simulink model "AT_power_supply"  (R2017a)
settings: Solver=VariableStepDiscrete  StartTime=0.0  StopTime=10.0  MaxStep=1e-4  RelTol=1e-3
model workspace (MAT data in the model file):
  C = [1.22730985268e-11  -9.79032554766e-13  -3.3876063565e-12  -2.00231039085e-12  -3.89359662643e-13  -1.2256864147e-12; -9.79032554766e-13  8.8541386421e-12  -3.48812783487e-12  -6.7988448902e-13  -2.32120771084e-13  -3.75147725397e-13; -3.3876063565e-12  -3.48812783487e-12  5.05683717303e-11  -4.82296810228e-13  -4.29846925887e-14  -1.14861569096e-12; -2.00231039085e-12  -6.7988448902e-13  -4.82296810228e-13  1.2217542164e-11  -1.06668598412e-12  -3.29793326195e-12; -3.89359662643e-13  -2.32120771084e-13  -4.29846925887e-14  -1.06668598412e-12  8.80500883356e-12  -3.55300206066e-12; -1.2256864147e-12  -3.75147725397e-13  -1.14861569096e-12  -3.29793326195e-12  -3.55300206066e-12  5.14882367603e-11]
  L = [0.00187555920474  0.00102764893826  0.00103076007408  0.00104087588335  0.000916441165262  0.00094103834573; 0.00102764893826  0.00220486482933  0.0010632014985  0.000914578394203  0.000842167961305  0.000853030250716; 0.00103076007408  0.0010632014985  0.00138127517435  0.000946699228346  0.000884811406268  0.000952474726801; 0.00104087588335  0.000914578394203  0.000946699228346  0.0018795120154  0.0010307312193  0.00103493155019; 0.000916441165262  0.000842167961305  0.000884811406268  0.0010307312193  0.00220867896719  0.00106461641191; 0.00094103834573  0.000853030250716  0.000952474726801  0.00103493155019  0.00106461641191  0.00136582310124]
  X = [0.589224301899  0.322845435491  0.323822827633  0.327000802842  0.287908483223  0.295635915369; 0.322845435491  0.692678715  0.334014601697  0.287323276436  0.264574868032  0.267987356894; 0.323822827633  0.334014601697  0.433940394034  0.297414334093  0.277971701374  0.299228760445; 0.327000802842  0.287323276436  0.297414334093  0.590466113991  0.323813762639  0.325133335506; 0.287908483223  0.264574868032  0.277971701374  0.323813762639  0.693876961748  0.334459109856; 0.295635915369  0.267987356894  0.299228760445  0.325133335506  0.334459109856  0.429085982097]
libraries: powerlib x20
settings Model: Creator=Administrator  LastModifiedBy=Administrator
settings DebuggingCC: UnconnectedInputMsg=none  UnconnectedOutputMsg=none  UnconnectedLineMsg=none

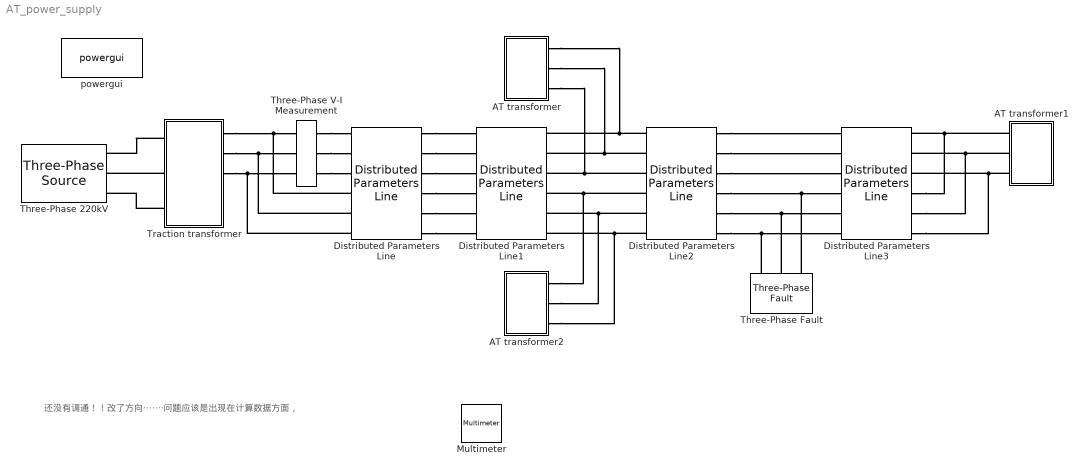
== system AT_power_supply ==
  note: 还没有调通！！改了方向·······问题应该是出现在计算数据方面，
  AT transformer : Subsystem
  AT transformer1 : Subsystem
  AT transformer2 : Subsystem
  Distributed Parameters Line : powerlib/Elements/Distributed Parameters Line  Phases=6  Frequency=50  Resistance=X  Inductance=L  Capacitance=C  Length=100  x1=[0 0 0 0; 0.0001244 0 0 0; 0.0002488 0 0 0; 0.0003733 0 0 0; 0.0004977 0 0 0; 0.0006221 0 0 0]  x2=[0 0 0 0; 0.0001244 0 0 0; 0.0002488 0 0 0; 0.0003733 0 0 0; 0.0004977 0 0 0; 0.0006221 0 0 0]  x3=[0 0 0 0; 0.0001244 0 0 0; 0.0002488 0 0 0; 0.0003733 0 0 0; 0.0004977 0 0 0; 0.0006221 0 0 0]  x4=[0 0 0 0; 0.0001244 0 0 0; 0.0002488 0 0 0; 0.0003733 0 0 0; 0.0004977 0 0 0; 0.0006221 0 0 0]  x5=0  V1=ones(3,3)  V2=ones(3,3)  I1=ones(3,3)  I2=ones(3,3)  nHarmo=1  Measurements=Phase-to-ground voltages
      settings: SourceProductName=Simscape Power Systems
  Distributed Parameters Line1 : powerlib/Elements/Distributed Parameters Line  Phases=6  Frequency=50  Resistance=X  Inductance=L  Capacitance=C  Length=10  x1=[0 0 0 0; 0.0001244 0 0 0; 0.0002488 0 0 0; 0.0003733 0 0 0; 0.0004977 0 0 0; 0.0006221 0 0 0]  x2=[0 0 0 0; 0.0001244 0 0 0; 0.0002488 0 0 0; 0.0003733 0 0 0; 0.0004977 0 0 0; 0.0006221 0 0 0]  x3=[0 0 0 0; 0.0001244 0 0 0; 0.0002488 0 0 0; 0.0003733 0 0 0; 0.0004977 0 0 0; 0.0006221 0 0 0]  x4=[0 0 0 0; 0.0001244 0 0 0; 0.0002488 0 0 0; 0.0003733 0 0 0; 0.0004977 0 0 0; 0.0006221 0 0 0]  x5=0  V1=ones(3,3)  V2=ones(3,3)  I1=ones(3,3)  I2=ones(3,3)  nHarmo=1  Measurements=None
      settings: SourceProductName=Simscape Power Systems
  Distributed Parameters Line2 : powerlib/Elements/Distributed Parameters Line  Phases=6  Frequency=50  Resistance=X  Inductance=L  Capacitance=C  Length=10  x1=[0 0 0 0; 0.0001244 0 0 0; 0.0002488 0 0 0; 0.0003733 0 0 0; 0.0004977 0 0 0; 0.0006221 0 0 0]  x2=[0 0 0 0; 0.0001244 0 0 0; 0.0002488 0 0 0; 0.0003733 0 0 0; 0.0004977 0 0 0; 0.0006221 0 0 0]  x3=[0 0 0 0; 0.0001244 0 0 0; 0.0002488 0 0 0; 0.0003733 0 0 0; 0.0004977 0 0 0; 0.0006221 0 0 0]  x4=[0 0 0 0; 0.0001244 0 0 0; 0.0002488 0 0 0; 0.0003733 0 0 0; 0.0004977 0 0 0; 0.0006221 0 0 0]  x5=0  V1=ones(3,3)  V2=ones(3,3)  I1=ones(3,3)  I2=ones(3,3)  nHarmo=1  Measurements=None
      settings: SourceProductName=Simscape Power Systems
  Distributed Parameters Line3 : powerlib/Elements/Distributed Parameters Line  Phases=6  Frequency=50  Resistance=X  Inductance=L  Capacitance=C  Length=10  x1=[0 0 0 0; 0.0001244 0 0 0; 0.0002488 0 0 0; 0.0003733 0 0 0; 0.0004977 0 0 0; 0.0006221 0 0 0]  x2=[0 0 0 0; 0.0001244 0 0 0; 0.0002488 0 0 0; 0.0003733 0 0 0; 0.0004977 0 0 0; 0.0006221 0 0 0]  x3=[0 0 0 0; 0.0001244 0 0 0; 0.0002488 0 0 0; 0.0003733 0 0 0; 0.0004977 0 0 0; 0.0006221 0 0 0]  x4=[0 0 0 0; 0.0001244 0 0 0; 0.0002488 0 0 0; 0.0003733 0 0 0; 0.0004977 0 0 0; 0.0006221 0 0 0]  x5=0  V1=ones(3,3)  V2=ones(3,3)  I1=ones(3,3)  I2=ones(3,3)  nHarmo=1  Measurements=None
      settings: SourceProductName=Simscape Power Systems
  Multimeter : powerlib/Measurements/Multimeter  PhasorSimulation=off  OutputType=Complex  sel=1  L=1  Gain=0  yselected={}  PSBOutputType=1  PSBequivalent=0  AxesSetting=[0,0.1,-100,100]  Display=0  SavedBlockNames=-11
  Three-Phase V-I Measurement : powerlib/Measurements/Three-Phase V-I Measurement  VoltageMeasurement=phase-to-ground  SetLabelV=on  LabelV=Vabc  Vpu=off  VpuLL=off  CurrentMeasurement=yes  SetLabelI=on  LabelI=Iabc  Ipu=off  Pbase=100e6  Vbase=500e3  OutputType=Complex  PhasorSimulation=off  PSBequivalent=0
  Three-Phase 220kV : powerlib/Electrical Sources/Three-Phase Source  InternalConnection=Yg  VoltagePhases=off  Voltage=220e3  PhaseAngle=0  Voltage_phases=[25e3 25e3 25e3]/sqrt(3)  PhaseAngles_phases=[0 -120 +120]  Frequency=50  NonIdealSource=on  SpecifyImpedance=on  Resistance=0.8929  Inductance=16.58e-3  ShortCircuitLevel=4e9  BaseVoltage=220e3  XRratio=16  BusType=swing  Pref=10e3  Qref=0  Prefabc=[10e3, 10e3, 10e3]  Qrefabc=[0, 0, 0]  Qmin=-inf  Qmax=inf
  Three-Phase Fault : powerlib/Elements/Three-Phase Fault  InitialStates=0  FaultA=on  FaultB=off  FaultC=off  GroundFault=on  SwitchTimes="[1/60  5/60]"  External=off  SwitchStatus=NaN  FaultResistance=0.001  GroundResistance=0.01  SnubberResistance=1e6  SnubberCapacitance=inf  Measurements=None
  Traction transformer : Subsystem
  powergui : powerlib/powergui  Priority=1  SimulationMode=Continuous  SampleTime=1e-6  frequency=60  Iterations=50  frequencyindice=60  Pbase=100e6  ErrMax=1e-4  UnitsV=kV  UnitsW=MW  buscounter=0  FunctionMessages=off  echomessages=off  EnableUseOfTLC=off  CurrentSourceSwitches=off  DisableSnubberDevices=off  DisableRonSwitches=off  DisableVfSwitches=off  DisplayEquations=off  SolverType=Tustin/Backward Euler (TBE)  Interpol=off  ExternalGateDelay=off  methode=off  Ts=100  x0status=blocks  SPID=on  SwTol=0  HookPort=off  RestoreLinks=warning  ResistiveCurrentMeasurement=off  Frange=[0:2:500]  Ylog=off  Xlog=on  ShowGrid=off  save=off  variable=ZData  structure=0  ZoomFFT=off  StartTime=0.0  cycles=1  DisplayStyle=1  fundamental=60  FreqAxis=off  MaxFrequency=1000  frequencyindicesteady=1  RmsSteady=1  display=off
  connections:
  Traction transformer/LConn2 -- Three-Phase 220kV/RConn2
  Traction transformer/LConn1 -- Three-Phase 220kV/RConn1
  Traction transformer/LConn3 -- Three-Phase 220kV/RConn3
  Distributed Parameters Line/RConn1 -- Distributed Parameters Line1/LConn1
  Distributed Parameters Line/RConn2 -- Distributed Parameters Line1/LConn2
  Distributed Parameters Line/RConn3 -- Distributed Parameters Line1/LConn3
  Distributed Parameters Line/RConn4 -- Distributed Parameters Line1/LConn4
  Distributed Parameters Line/RConn5 -- Distributed Parameters Line1/LConn5
  Distributed Parameters Line/RConn6 -- Distributed Parameters Line1/LConn6
  Distributed Parameters Line2/LConn1 -- AT transformer/RConn1 -- Distributed Parameters Line1/RConn1
  Distributed Parameters Line2/LConn2 -- AT transformer/RConn2 -- Distributed Parameters Line1/RConn2
  Distributed Parameters Line2/LConn3 -- AT transformer/RConn3 -- Distributed Parameters Line1/RConn3
  Distributed Parameters Line2/LConn4 -- AT transformer2/RConn1 -- Distributed Parameters Line1/RConn4
  Distributed Parameters Line2/LConn5 -- AT transformer2/RConn2 -- Distributed Parameters Line1/RConn5
  Distributed Parameters Line2/LConn6 -- AT transformer2/RConn3 -- Distributed Parameters Line1/RConn6
  Distributed Parameters Line2/RConn1 -- Distributed Parameters Line3/LConn1
  Distributed Parameters Line2/RConn2 -- Distributed Parameters Line3/LConn2
  Distributed Parameters Line2/RConn3 -- Distributed Parameters Line3/LConn3
  Distributed Parameters Line2/RConn4 -- Three-Phase Fault/LConn1 -- Distributed Parameters Line3/LConn4
  Distributed Parameters Line2/RConn5 -- Three-Phase Fault/LConn2 -- Distributed Parameters Line3/LConn5
  Distributed Parameters Line2/RConn6 -- Three-Phase Fault/LConn3 -- Distributed Parameters Line3/LConn6
  AT transformer1/RConn1 -- Distributed Parameters Line3/RConn4 -- Distributed Parameters Line3/RConn1
  AT transformer1/RConn2 -- Distributed Parameters Line3/RConn5 -- Distributed Parameters Line3/RConn2
  AT transformer1/RConn3 -- Distributed Parameters Line3/RConn6 -- Distributed Parameters Line3/RConn3
  Traction transformer/RConn1 -- Distributed Parameters Line/LConn4 -- Three-Phase V-I Measurement/LConn1
  Traction transformer/RConn2 -- Distributed Parameters Line/LConn5 -- Three-Phase V-I Measurement/LConn2
  Traction transformer/RConn3 -- Distributed Parameters Line/LConn6 -- Three-Phase V-I Measurement/LConn3
  Three-Phase V-I Measurement/RConn1 -- Distributed Parameters Line/LConn1
  Three-Phase V-I Measurement/RConn2 -- Distributed Parameters Line/LConn2
  Three-Phase V-I Measurement/RConn3 -- Distributed Parameters Line/LConn3

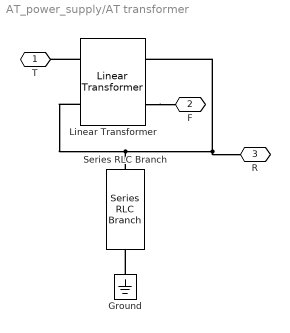
== system AT_power_supply/AT transformer ==
  Ground : powerlib/Elements/Ground  LConnTagsString=a
  Linear Transformer : powerlib/Elements/Linear Transformer  UNITS=pu  NominalPower=[ 32e6 50 ]  winding1="[ 27.5e3  0.002  0.08 ]"  winding2="[ 27.5e3  0.002  0.08 ]"  ThreeWindings=off  winding3=[ 315e3 0.002 0.08 ]  RmLm=[ 500 500 ]  Measurements=All voltages and currents  DataType=off
  Series RLC Branch : powerlib/Elements/Series RLC Branch  LConnTagsString=__new0  RConnTagsString=__new0  BranchType=R  Resistance=0.42  Inductance=1e-3  SetiL0=off  InitialCurrent=0  Capacitance=1e-6  Setx0=off  InitialVoltage=0  Measurements=None
  T : PMIOPort  Port=1  Side=Right
  F : PMIOPort  Port=2  Side=Right
  R : PMIOPort  Port=3  Side=Right
  connections:
  Linear Transformer/RConn2 -- F/RConn1
  Linear Transformer/LConn1 -- T/RConn1
  Ground/LConn1 -- Series RLC Branch/RConn1
  Linear Transformer/LConn2 -- Series RLC Branch/LConn1 -- R/RConn1 -- Linear Transformer/RConn1

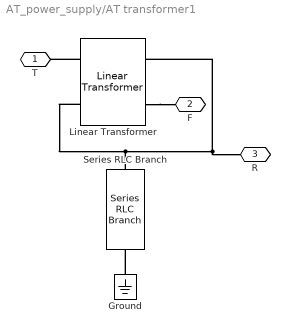
== system AT_power_supply/AT transformer1 ==
  Ground : powerlib/Elements/Ground  LConnTagsString=a
  Linear Transformer : powerlib/Elements/Linear Transformer  UNITS=pu  NominalPower=[ 32e6 50 ]  winding1="[ 27.5e3  0.002  0.08 ]"  winding2="[ 27.5e3  0.002  0.08 ]"  ThreeWindings=off  winding3=[ 315e3 0.002 0.08 ]  RmLm=[ 500 500 ]  Measurements=All voltages and currents  DataType=off
  Series RLC Branch : powerlib/Elements/Series RLC Branch  LConnTagsString=__new0  RConnTagsString=__new0  BranchType=R  Resistance=0.42  Inductance=1e-3  SetiL0=off  InitialCurrent=0  Capacitance=1e-6  Setx0=off  InitialVoltage=0  Measurements=None
  T : PMIOPort  Port=1  Side=Right
  F : PMIOPort  Port=2  Side=Right
  R : PMIOPort  Port=3  Side=Right
  connections:
  Linear Transformer/RConn2 -- F/RConn1
  Linear Transformer/LConn1 -- T/RConn1
  Ground/LConn1 -- Series RLC Branch/RConn1
  Linear Transformer/LConn2 -- Series RLC Branch/LConn1 -- R/RConn1 -- Linear Transformer/RConn1

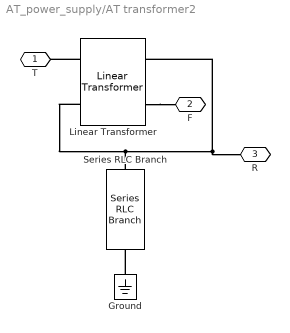
== system AT_power_supply/AT transformer2 ==
  Ground : powerlib/Elements/Ground  LConnTagsString=a
  Linear Transformer : powerlib/Elements/Linear Transformer  UNITS=pu  NominalPower=[ 32e6 50 ]  winding1="[ 27.5e3  0.002  0.08 ]"  winding2="[ 27.5e3  0.002  0.08 ]"  ThreeWindings=off  winding3=[ 315e3 0.002 0.08 ]  RmLm=[ 500 500 ]  Measurements=All voltages and currents  DataType=off
  Series RLC Branch : powerlib/Elements/Series RLC Branch  LConnTagsString=__new0  RConnTagsString=__new0  BranchType=R  Resistance=0.42  Inductance=1e-3  SetiL0=off  InitialCurrent=0  Capacitance=1e-6  Setx0=off  InitialVoltage=0  Measurements=None
  T : PMIOPort  Port=1  Side=Right
  F : PMIOPort  Port=2  Side=Right
  R : PMIOPort  Port=3  Side=Right
  connections:
  Linear Transformer/RConn2 -- F/RConn1
  Linear Transformer/LConn1 -- T/RConn1
  Ground/LConn1 -- Series RLC Branch/RConn1
  Linear Transformer/LConn2 -- Series RLC Branch/LConn1 -- R/RConn1 -- Linear Transformer/RConn1

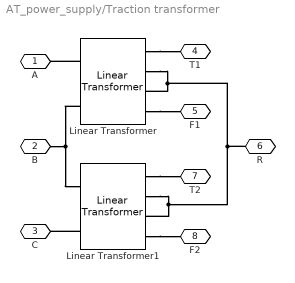
== system AT_power_supply/Traction transformer ==
  Linear Transformer : powerlib/Elements/Linear Transformer  UNITS=pu  NominalPower=[ 25e6 50 ]  winding1="[ 220e3  0.002  0.08 ]"  winding2="[ 27.5e3  0.002  0.08 ]"  ThreeWindings=on  winding3=[ 27.5e3 0.002 0.08 ]  RmLm=[ 500 500 ]  Measurements=All voltages and currents  DataType=off
  Linear Transformer1 : powerlib/Elements/Linear Transformer  UNITS=pu  NominalPower=[ 25e6 50 ]  winding1="[ 220e3  0.002  0.08 ]"  winding2="[ 27.5e3  0.002  0.08 ]"  ThreeWindings=on  winding3=[ 27.5e3 0.002 0.08 ]  RmLm=[ 500 500 ]  Measurements=All voltages and currents  DataType=off
  A : PMIOPort  Port=1  Side=Left
  B : PMIOPort  Port=2  Side=Left
  C : PMIOPort  Port=3  Side=Left
  T1 : PMIOPort  Port=4  Side=Right
  F1 : PMIOPort  Port=5  Side=Right
  R : PMIOPort  Port=6  Side=Right
  T2 : PMIOPort  Port=7  Side=Right
  F2 : PMIOPort  Port=8  Side=Right
  connections:
  Linear Transformer/LConn2 -- B/RConn1 -- Linear Transformer1/LConn1
  Linear Transformer1/RConn2 -- R/RConn1 -- Linear Transformer/RConn2 -- Linear Transformer/RConn3 -- Linear Transformer1/RConn3
  Linear Transformer/RConn1 -- T1/RConn1
  Linear Transformer1/RConn1 -- T2/RConn1
  Linear Transformer/RConn4 -- F1/RConn1
  Linear Transformer/LConn1 -- A/RConn1
  Linear Transformer1/LConn2 -- C/RConn1
  Linear Transformer1/RConn4 -- F2/RConn1
